simulink model "Project_Simulation_Case_1"  (R2018b)
settings: Solver=VariableStepAuto  StartTime=0.0  StopTime=60  FixedStep=0.0001  RelTol=1e-3
InitFcn:
  | Initial_Data_Case_1
StopFcn:
  | Plots_Case_1
undefined symbols (not defined in the file or in its folder): alpha1, alpha2, alpha3, c1, c2, c3, gamma_t, landa1, landa2, landa3, Vg_t, zita_t
settings Model: Creator=User  LastModifiedBy=User

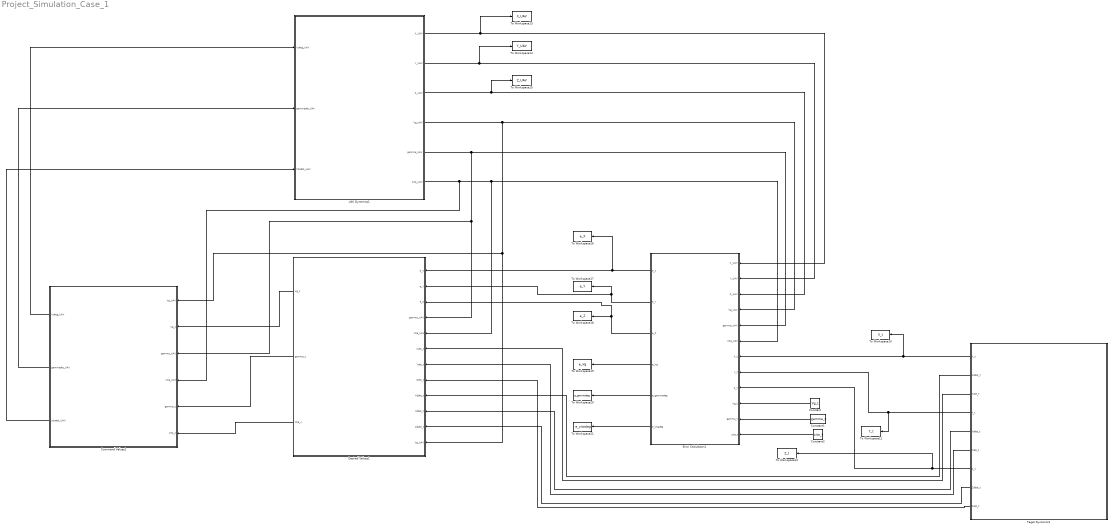
== system Project_Simulation_Case_1 ==
  Command Values1 : Subsystem
  Constant : Constant  Value=Vg_t
  Constant1 : Constant  Value=gamma_t
  Constant2 : Constant  Value=zita_t
  Desired Values1 : Subsystem
  Error Calculation1 : MATLAB Function  TreatAsAtomicUnit=on
  Taget Dynamics1 : Subsystem
  To Workspace10 : ToWorkspace  VariableName=X_t  SaveFormat=Timeseries  SampleTime=-1
  To Workspace11 : ToWorkspace  VariableName=Y_t  SaveFormat=Timeseries  SampleTime=-1
  To Workspace12 : ToWorkspace  VariableName=Z_t  SaveFormat=Timeseries  SampleTime=-1
  To Workspace13 : ToWorkspace  VariableName=X_UAV  SaveFormat=Timeseries  SampleTime=-1
  To Workspace14 : ToWorkspace  VariableName=Y_UAV  SaveFormat=Timeseries  SampleTime=-1
  To Workspace15 : ToWorkspace  VariableName=Z_UAV  SaveFormat=Timeseries  SampleTime=-1
  To Workspace16 : ToWorkspace  VariableName=e_X  SaveFormat=Timeseries  SampleTime=-1
  To Workspace17 : ToWorkspace  VariableName=e_Y  SaveFormat=Timeseries  SampleTime=-1
  To Workspace18 : ToWorkspace  VariableName=e_Z  SaveFormat=Timeseries  SampleTime=-1
  To Workspace19 : ToWorkspace  VariableName=e_Vg  SaveFormat=Timeseries  SampleTime=-1
  To Workspace20 : ToWorkspace  VariableName=e_gammadeg  SaveFormat=Timeseries  SampleTime=-1
  To Workspace21 : ToWorkspace  VariableName=e_zitadeg  SaveFormat=Timeseries  SampleTime=-1
  UAV Dynamics1 : Subsystem
  wires:
  Taget Dynamics1/4(Y_t) -> To Workspace11/1, Error Calculation1/8(Y_t)
  Taget Dynamics1/8(Zddot_t) -> Desired Values1/11(Zddot_t)
  UAV Dynamics1/4(Vg_UAV) -> Command Values1/1(Vg_UAV), Desired Values1/12(Vg_UAV), Error Calculation1/4(Vg_UAV)
  Error Calculation1/3(e_Z) -> Desired Values1/3(e_Z), To Workspace18/1
  Error Calculation1/4(e_Vg) -> To Workspace19/1
  Command Values1/1(Vdotg_UAV) -> UAV Dynamics1/1(Vdotg_UAV)
  Command Values1/3(zitadot_UAV) -> UAV Dynamics1/3(zitadot_UAV)
  Taget Dynamics1/7(Z_t) -> To Workspace12/1, Error Calculation1/9(Z_t)
  Taget Dynamics1/3(Xdot_t) -> Desired Values1/6(Xdot_t)
  Desired Values1/1(Vg_c) -> Command Values1/2(Vg_c)
  Taget Dynamics1/1(X_t) -> To Workspace10/1, Error Calculation1/7(X_t)
  UAV Dynamics1/6(zita_UAV) -> Command Values1/4(zita_UAV), Error Calculation1/6(zita_UAV), Desired Values1/5(zita_UAV)
  Command Values1/2(gammadot_UAV) -> UAV Dynamics1/2(gammadot_UAV)
  Error Calculation1/6(e_zitadeg) -> To Workspace21/1
  Taget Dynamics1/6(Ydot_t) -> Desired Values1/7(Ydot_t)
  UAV Dynamics1/5(gamma_UAV) -> Desired Values1/4(gamma_UAV), Command Values1/3(gamma_UAV), Error Calculation1/5(gamma_UAV)
  Taget Dynamics1/9(Zdot_t) -> Desired Values1/8(Zdot_t)
  UAV Dynamics1/1(X_UAV) -> To Workspace13/1, Error Calculation1/1(X_UAV)
  Taget Dynamics1/2(Xddot_t) -> Desired Values1/9(Xddot_t)
  UAV Dynamics1/2(Y_UAV) -> To Workspace14/1, Error Calculation1/2(Y_UAV)
  Taget Dynamics1/5(Yddot_t) -> Desired Values1/10(Yddot_t)
  Error Calculation1/5(e_gammadeg) -> To Workspace20/1
  Error Calculation1/2(e_Y) -> Desired Values1/2(e_Y), To Workspace17/1
  Constant/1 -> Error Calculation1/10(Vg_t)
  Error Calculation1/1(e_X) -> Desired Values1/1(e_X), To Workspace16/1
  UAV Dynamics1/3(Z_UAV) -> To Workspace15/1, Error Calculation1/3(Z_UAV)
  Constant2/1 -> Error Calculation1/12(zita_t)
  Constant1/1 -> Error Calculation1/11(gamma_t)
  Desired Values1/2(gamma_c) -> Command Values1/5(gamma_c)
  Desired Values1/3(zita_c) -> Command Values1/6(zita_c)

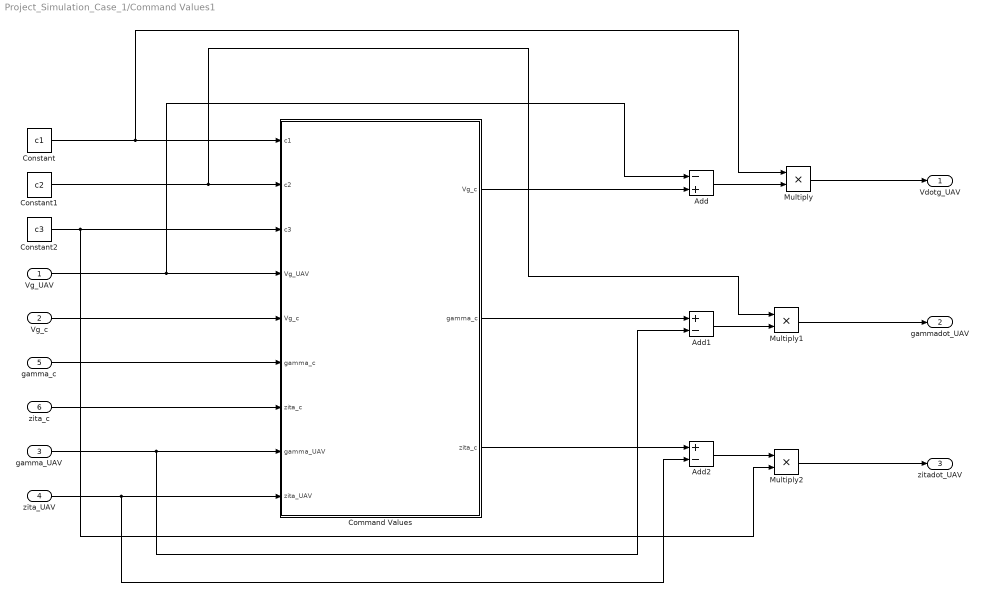
== system Project_Simulation_Case_1/Command Values1 ==
  Vg_UAV : Inport
  Vg_c : Inport  Port=2
  gamma_UAV : Inport  Port=3
  zita_UAV : Inport  Port=4
  gamma_c : Inport  Port=5
  zita_c : Inport  Port=6
  Add : Sum  Inputs=-+
  Add1 : Sum  Inputs=+-
  Add2 : Sum  Inputs=+-
  Command Values : MATLAB Function  TreatAsAtomicUnit=on
  Constant : Constant  Value=c1
  Constant1 : Constant  Value=c2
  Constant2 : Constant  Value=c3
  Multiply : Product
  Multiply1 : Product
  Multiply2 : Product
  Vdotg_UAV : Outport
  gammadot_UAV : Outport  Port=2
  zitadot_UAV : Outport  Port=3
  wires:
  Command Values/2(gamma_c) -> Add1/1
  Command Values/3(zita_c) -> Add2/1
  Vg_UAV/1 -> Add/1, Command Values/4(Vg_UAV)
  Vg_c/1 -> Command Values/5("Vg_c ")
  Constant/1 -> Multiply/1, Command Values/1(c1)
  Constant1/1 -> Multiply1/1, Command Values/2(c2)
  Constant2/1 -> Command Values/3(c3), Multiply2/2
  gamma_UAV/1 -> Add1/2, Command Values/8(gamma_UAV)
  zita_UAV/1 -> Add2/2, Command Values/9(zita_UAV)
  Multiply/1 -> Vdotg_UAV/1
  Multiply1/1 -> gammadot_UAV/1
  Multiply2/1 -> zitadot_UAV/1
  Command Values/1(Vg_c) -> Add/2
  Add/1 -> Multiply/2
  Add1/1 -> Multiply1/2
  Add2/1 -> Multiply2/1
  zita_c/1 -> Command Values/7("zita_c ")
  gamma_c/1 -> Command Values/6("gamma_c ")

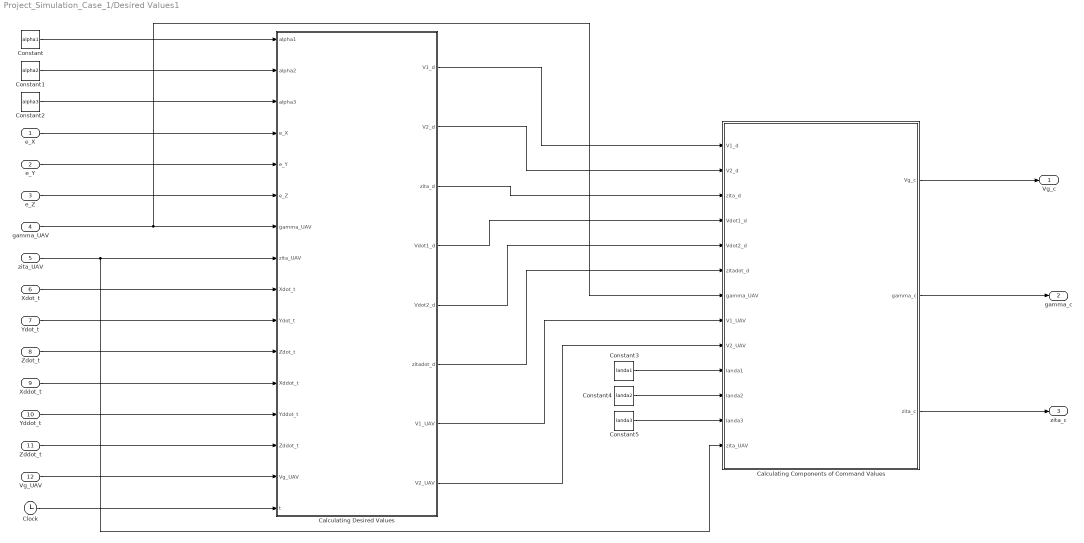
== system Project_Simulation_Case_1/Desired Values1 ==
  e_X : Inport
  e_Y : Inport  Port=2
  e_Z : Inport  Port=3
  gamma_UAV : Inport  Port=4
  zita_UAV : Inport  Port=5
  Xdot_t : Inport  Port=6
  Ydot_t : Inport  Port=7
  Zdot_t : Inport  Port=8
  Xddot_t : Inport  Port=9
  Yddot_t : Inport  Port=10
  Zddot_t : Inport  Port=11
  Vg_UAV : Inport  Port=12
  Calculating Components of Command Values : MATLAB Function  TreatAsAtomicUnit=on
  Calculating Desired Values : MATLAB Function  TreatAsAtomicUnit=on
  Clock : Clock
  Constant : Constant  Value=alpha1
  Constant1 : Constant  Value=alpha2
  Constant2 : Constant  Value=alpha3
  Constant3 : Constant  Value=landa1
  Constant4 : Constant  Value=landa2
  Constant5 : Constant  Value=landa3
  Vg_c : Outport
  gamma_c : Outport  Port=2
  zita_c : Outport  Port=3
  wires:
  Constant/1 -> Calculating Desired Values/1(alpha1)
  Constant1/1 -> Calculating Desired Values/2(alpha2)
  Constant2/1 -> Calculating Desired Values/3(alpha3)
  e_X/1 -> Calculating Desired Values/4(e_X)
  e_Y/1 -> Calculating Desired Values/5(e_Y)
  e_Z/1 -> Calculating Desired Values/6(e_Z)
  gamma_UAV/1 -> Calculating Components of Command Values/7(gamma_UAV), Calculating Desired Values/7(gamma_UAV)
  zita_UAV/1 -> Calculating Components of Command Values/13(zita_UAV), Calculating Desired Values/8(zita_UAV)
  Xdot_t/1 -> Calculating Desired Values/9(Xdot_t)
  Ydot_t/1 -> Calculating Desired Values/10(Ydot_t)
  Zdot_t/1 -> Calculating Desired Values/11(Zdot_t)
  Xddot_t/1 -> Calculating Desired Values/12(Xddot_t)
  Yddot_t/1 -> Calculating Desired Values/13(Yddot_t)
  Zddot_t/1 -> Calculating Desired Values/14(Zddot_t)
  Vg_UAV/1 -> Calculating Desired Values/15(Vg_UAV)
  Calculating Desired Values/1(V1_d) -> Calculating Components of Command Values/1(V1_d)
  Calculating Desired Values/2(V2_d) -> Calculating Components of Command Values/2(V2_d)
  Calculating Desired Values/3(zita_d) -> Calculating Components of Command Values/3(zita_d)
  Calculating Desired Values/4(Vdot1_d) -> Calculating Components of Command Values/4(Vdot1_d)
  Calculating Desired Values/5(Vdot2_d) -> Calculating Components of Command Values/5(Vdot2_d)
  Calculating Desired Values/6(zitadot_d) -> Calculating Components of Command Values/6(zitadot_d)
  Calculating Desired Values/7(V1_UAV) -> Calculating Components of Command Values/8(V1_UAV)
  Calculating Desired Values/8(V2_UAV) -> Calculating Components of Command Values/9(V2_UAV)
  Constant3/1 -> Calculating Components of Command Values/10(landa1)
  Constant4/1 -> Calculating Components of Command Values/11(landa2)
  Constant5/1 -> Calculating Components of Command Values/12(landa3)
  Calculating Components of Command Values/1(Vg_c) -> Vg_c/1
  Calculating Components of Command Values/2(gamma_c) -> gamma_c/1
  Calculating Components of Command Values/3(zita_c) -> zita_c/1
  Clock/1 -> Calculating Desired Values/16(t)

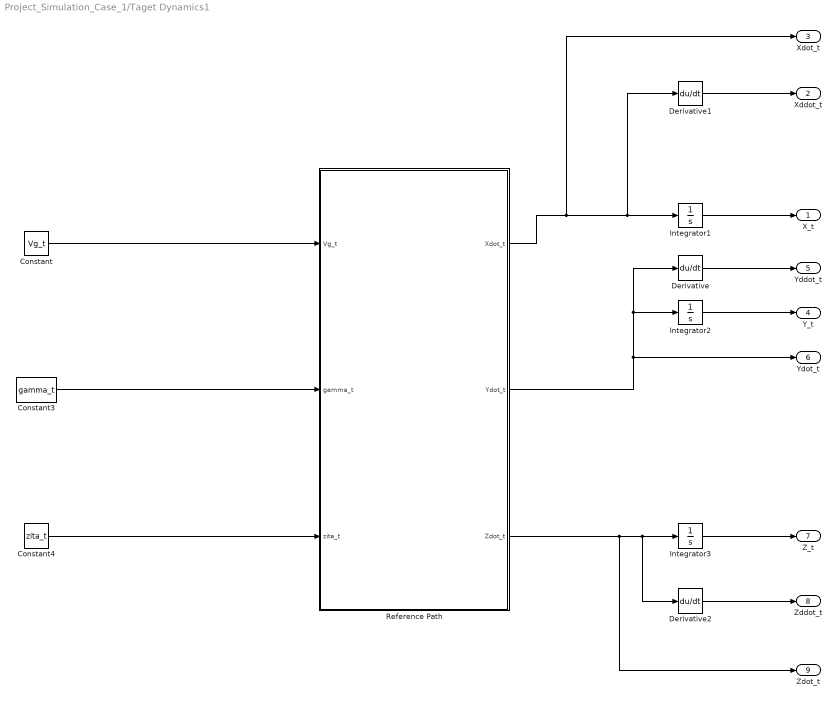
== system Project_Simulation_Case_1/Taget Dynamics1 ==
  Constant : Constant  Value=Vg_t
  Constant3 : Constant  Value=gamma_t
  Constant4 : Constant  Value=zita_t
  Derivative : Derivative
  Derivative1 : Derivative
  Derivative2 : Derivative
  Integrator1 : Integrator  InitialCondition=100
  Integrator2 : Integrator  InitialCondition=100
  Integrator3 : Integrator  InitialCondition=100
  Reference Path : MATLAB Function  TreatAsAtomicUnit=on
  X_t : Outport
  Xddot_t : Outport  Port=2
  Xdot_t : Outport  Port=3
  Y_t : Outport  Port=4
  Yddot_t : Outport  Port=5
  Ydot_t : Outport  Port=6
  Z_t : Outport  Port=7
  Zddot_t : Outport  Port=8
  Zdot_t : Outport  Port=9
  wires:
  Integrator1/1 -> X_t/1
  Derivative1/1 -> Xddot_t/1
  Reference Path/1(Xdot_t) -> Derivative1/1, Integrator1/1, Xdot_t/1
  Integrator2/1 -> Y_t/1
  Reference Path/2(Ydot_t) -> Integrator2/1, Derivative/1, Ydot_t/1
  Derivative/1 -> Yddot_t/1
  Reference Path/3(Zdot_t) -> Zdot_t/1, Derivative2/1, Integrator3/1
  Derivative2/1 -> Zddot_t/1
  Integrator3/1 -> Z_t/1
  Constant/1 -> Reference Path/1(Vg_t)
  Constant3/1 -> Reference Path/2(gamma_t)
  Constant4/1 -> Reference Path/3(zita_t)

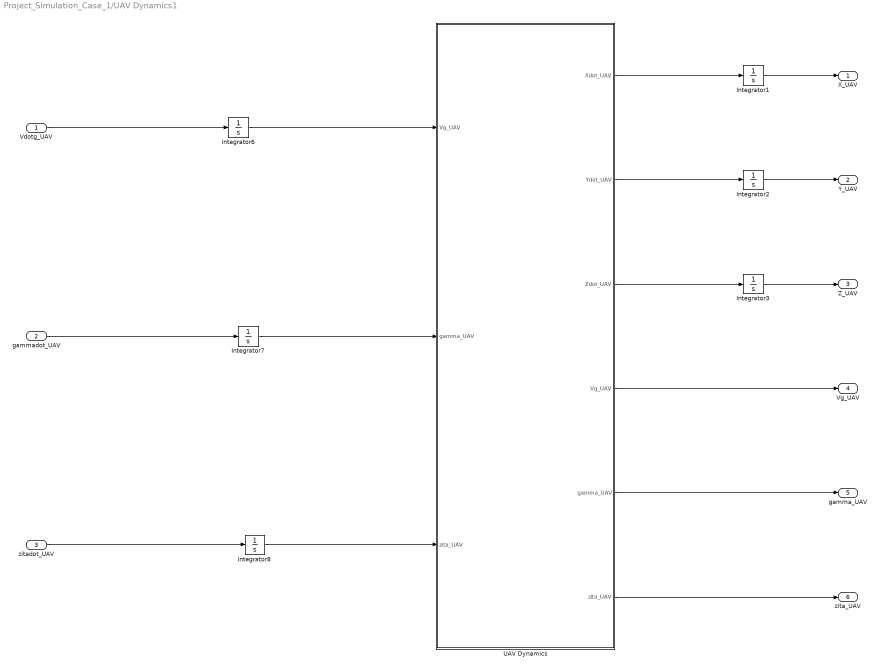
== system Project_Simulation_Case_1/UAV Dynamics1 ==
  Vdotg_UAV : Inport
  gammadot_UAV : Inport  Port=2
  zitadot_UAV : Inport  Port=3
  Integrator1 : Integrator  InitialCondition=80
  Integrator2 : Integrator  InitialCondition=90
  Integrator3 : Integrator  InitialCondition=70
  Integrator6 : Integrator  InitialCondition=8
  Integrator7 : Integrator  InitialCondition=0*pi/180
  Integrator8 : Integrator  InitialCondition=0*pi/180
  UAV Dynamics : MATLAB Function  TreatAsAtomicUnit=on
  X_UAV : Outport
  Y_UAV : Outport  Port=2
  Z_UAV : Outport  Port=3
  Vg_UAV : Outport  Port=4
  gamma_UAV : Outport  Port=5
  zita_UAV : Outport  Port=6
  wires:
  Integrator3/1 -> Z_UAV/1
  UAV Dynamics/1(Xdot_UAV) -> Integrator1/1
  Integrator2/1 -> Y_UAV/1
  UAV Dynamics/2(Ydot_UAV) -> Integrator2/1
  UAV Dynamics/3(Zdot_UAV) -> Integrator3/1
  Integrator1/1 -> X_UAV/1
  UAV Dynamics/4(Vg_UAV) -> Vg_UAV/1
  UAV Dynamics/5(gamma_UAV) -> gamma_UAV/1
  UAV Dynamics/6(zita_UAV) -> zita_UAV/1
  Vdotg_UAV/1 -> Integrator6/1
  Integrator6/1 -> UAV Dynamics/1("Vg_UAV ")
  gammadot_UAV/1 -> Integrator7/1
  Integrator7/1 -> UAV Dynamics/2("gamma_UAV ")
  zitadot_UAV/1 -> Integrator8/1
  Integrator8/1 -> UAV Dynamics/3("zita_UAV ")

== matlab function Project_Simulation_Case_1/Command Values1/Command Values ==
  data: c1 input; Vg_c output; c2 input; c3 input; Vg_UAV input; Vg_c input; gamma_c input; zita_c input; gamma_c output; zita_c output; gamma_UAV input; zita_UAV input
function [Vg_c,gamma_c,zita_c] = fcn(c1,c2,c3,Vg_UAV,Vg_c,gamma_c,zita_c,gamma_UAV,zita_UAV)

Vg_c = Vg_UAV - (1/c1)*(Vg_c);
gamma_c = gamma_UAV - (1/(c2*Vg_UAV))*(gamma_c);
zita_c = zita_UAV - (1/c3)*zita_c;

== matlab function Project_Simulation_Case_1/Desired Values1/Calculating Components of Command Values ==
  data: V1_d input; Vg_c output; V2_d input; zita_d input; Vdot1_d input; Vdot2_d input; zitadot_d input; gamma_UAV input; V1_UAV input; V2_UAV input; landa1 input; landa2 input; landa3 input; gamma_c output; zita_c output; zita_UAV input
function [Vg_c,gamma_c,zita_c] = fcn(V1_d,V2_d,zita_d,Vdot1_d,Vdot2_d,zitadot_d,gamma_UAV, V1_UAV,V2_UAV,landa1,landa2,landa3,zita_UAV)

Vg_c1 = -Vdot1_d + landa1*(V1_UAV - V1_d);
Vg_c2 = -Vdot2_d + landa2*(V2_UAV - V2_d);
Vg_c = Vg_c1*cos(gamma_UAV) + Vg_c2*sin(gamma_UAV);
gamma_c1 = -Vdot1_d + landa1*(V1_UAV - V1_d);
gamma_c2 = -Vdot2_d + landa2*(V2_UAV - V2_d);
gamma_c = -sin(gamma_UAV)*gamma_c1 + cos(gamma_UAV)*gamma_c2;
zita_c = -zitadot_d + landa3*(zita_UAV - zita_d);

== matlab function Project_Simulation_Case_1/Desired Values1/Calculating Desired Values ==
  data: alpha1 input; V1_d output; V2_d output; zita_d output; Vdot1_d output; Vdot2_d output; zitadot_d output; alpha2 input; alpha3 input; e_X input; e_Y input; e_Z input; gamma_UAV input; zita_UAV input; Xdot_t input; Ydot_t input; Zdot_t input; Xddot_t input; Yddot_t input; Zddot_t input; Vg_UAV input; V1_UAV output; V2_UAV output; t input
function [V1_d,V2_d,zita_d,Vdot1_d,Vdot2_d,zitadot_d,V1_UAV,V2_UAV] = fcn(alpha1,alpha2,alpha3,e_X,e_Y,e_Z,gamma_UAV,zita_UAV,Xdot_t,Ydot_t,Zdot_t,Xddot_t,Yddot_t,Zddot_t,Vg_UAV,t)

V1_UAV = Vg_UAV*cos(gamma_UAV);
V2_UAV = Vg_UAV*sin(gamma_UAV);
V1_d = sqrt((-alpha1*e_X + Xdot_t)^2 + (-alpha2*e_Y + Ydot_t)^2);
V2_d = -alpha3*e_Z + Zdot_t;
y = (-alpha2*e_Y + Ydot_t);
x = (-alpha1*e_X + Xdot_t);
zita_d = atan2(y,x);
Vdot1_d = (1/V1_d)*((-alpha1*e_X + Xdot_t)*(-alpha1*V1_UAV*cos(zita_UAV) + Xddot_t + alpha1*Xdot_t) + (-alpha2*e_Y + Ydot_t)*(-alpha2*V1_UAV*sin(zita_UAV) + Yddot_t + alpha2*Ydot_t));
Vdot2_d = -alpha3*V2_UAV + Zddot_t + alpha3*Zdot_t;
zitadot_d = (1/V1_d)*(cos(zita_d)*(-alpha2*V1_UAV*sin(zita_UAV) + Yddot_t + alpha2*Ydot_t) - sin(zita_d)*(-alpha1*V1_UAV*cos(zita_UAV) + Xddot_t + alpha1*Xdot_t));

== matlab function Project_Simulation_Case_1/Error Calculation1 ==
  data: X_UAV input; e_X output; Y_UAV input; Z_UAV input; Vg_UAV input; gamma_UAV input; zita_UAV input; X_t input; Y_t input; Z_t input; Vg_t input; gamma_t input; zita_t input; e_Y output; e_Z output; e_Vg output; e_gammadeg output; e_zitadeg output
function [e_X,e_Y,e_Z,e_Vg,e_gammadeg,e_zitadeg] = fcn(X_UAV,Y_UAV,Z_UAV,Vg_UAV,gamma_UAV,zita_UAV,X_t,Y_t,Z_t,Vg_t,gamma_t,zita_t)

e_X = X_UAV - X_t;
e_Y = Y_UAV - Y_t;
e_Z = Z_UAV - Z_t;
e_Vg = Vg_UAV - Vg_t;
e_gamma = gamma_UAV - gamma_t;
e_zita = zita_UAV - zita_t;
e_gammadeg = e_gamma*(180/pi);
e_zitadeg = e_zita*(180/pi);

== matlab function Project_Simulation_Case_1/Taget Dynamics1/Reference Path ==
  data: Vg_t input; Xdot_t output; gamma_t input; zita_t input; Ydot_t output; Zdot_t output
function [Xdot_t,Ydot_t,Zdot_t]  = fcn(Vg_t,gamma_t,zita_t)

Xdot_t = Vg_t*cos(gamma_t)*cos(zita_t);
Ydot_t = Vg_t*cos(gamma_t)*sin(zita_t);
Zdot_t = Vg_t*sin(gamma_t);

== matlab function Project_Simulation_Case_1/UAV Dynamics1/UAV Dynamics ==
  data: Xdot_UAV output; Ydot_UAV output; Vg_UAV input; Zdot_UAV output; gamma_UAV input; zita_UAV input; Vg_UAV output; gamma_UAV output; zita_UAV output
function [Xdot_UAV,Ydot_UAV,Zdot_UAV,Vg_UAV,gamma_UAV,zita_UAV]  = fcn(Vg_UAV,gamma_UAV,zita_UAV)

Xdot_UAV = Vg_UAV*cos(gamma_UAV)*cos(zita_UAV);
Ydot_UAV = Vg_UAV*cos(gamma_UAV)*sin(zita_UAV);
Zdot_UAV = Vg_UAV*sin(gamma_UAV);
